simulink model "test_ffts"  (Simulink 6.2)
settings: Solver=ode45  StartTime=0.0  StopTime=300  RelTol=1e-3
undefined symbols (not defined in the file or in its folder): now
libraries: xbsIndex_r3 x1135, fft_library x1, simulink x1
(part 11 of 15)

== system test_ffts/r4_dit_fft/quadplex_bitrev/biplex_bitrev0/bit_reverse ==
  in : Inport  Port=1  LatchInput=off
  bit0 : xbsIndex_r3/Slice  mode=Lower Bit Location + Width  nbits=1  bit1=0  base1=MSB of Input  bit0=0  base0=LSB of Input  boolean_output=off  explicit_period=off  period=1  dbl_ovrd=off
  bit1 : xbsIndex_r3/Slice  mode=Lower Bit Location + Width  nbits=1  bit1=0  base1=MSB of Input  bit0=1  base0=LSB of Input  boolean_output=off  explicit_period=off  period=1  dbl_ovrd=off
  bit2 : xbsIndex_r3/Slice  mode=Lower Bit Location + Width  nbits=1  bit1=0  base1=MSB of Input  bit0=2  base0=LSB of Input  boolean_output=off  explicit_period=off  period=1  dbl_ovrd=off
  bit3 : xbsIndex_r3/Slice  mode=Lower Bit Location + Width  nbits=1  bit1=0  base1=MSB of Input  bit0=3  base0=LSB of Input  boolean_output=off  explicit_period=off  period=1  dbl_ovrd=off
  concat : xbsIndex_r3/Concat  num_inputs=4  explicit_period=off  period=1  dbl_ovrd=off
  out : Outport
  wires:
  in/1 -> bit3/1, bit2/1, bit1/1, bit0/1
  bit3/1 -> concat/4
  bit2/1 -> concat/3
  bit1/1 -> concat/2
  bit0/1 -> concat/1
  concat/1 -> out/1

== system test_ffts/r4_dit_fft/quadplex_bitrev/biplex_bitrev0/c_to_ri ==
  c : Inport  Port=1  LatchInput=off
  force_im : xbsIndex_r3/Reinterpret  force_arith_type=on  arith_type="Signed  (2's comp)"  force_bin_pt=on  bin_pt=0  force_valid=on
  force_re : xbsIndex_r3/Reinterpret  force_arith_type=on  arith_type="Signed  (2's comp)"  force_bin_pt=on  bin_pt=0  force_valid=on
  slice_im : xbsIndex_r3/Slice  mode=Lower Bit Location + Width  nbits=14  bit1=0  base1=MSB of Input  bit0=0  base0=LSB of Input  boolean_output=off  explicit_period=off  period=1  dbl_ovrd=off
  slice_re : xbsIndex_r3/Slice  mode=Upper Bit Location + Width  nbits=14  bit1=0  base1=MSB of Input  bit0=0  base0=LSB of Input  boolean_output=off  explicit_period=off  period=1  dbl_ovrd=off
  re : Outport
  im : Outport  Port=2
  wires:
  slice_re/1 -> force_re/1
  slice_im/1 -> force_im/1
  force_re/1 -> re/1
  force_im/1 -> im/1
  c/1 -> slice_re/1, slice_im/1

== system test_ffts/r4_dit_fft/quadplex_bitrev/biplex_bitrev0/c_to_ri1 ==
  c : Inport  Port=1  LatchInput=off
  force_im : xbsIndex_r3/Reinterpret  force_arith_type=on  arith_type="Signed  (2's comp)"  force_bin_pt=on  bin_pt=0  force_valid=on
  force_re : xbsIndex_r3/Reinterpret  force_arith_type=on  arith_type="Signed  (2's comp)"  force_bin_pt=on  bin_pt=0  force_valid=on
  slice_im : xbsIndex_r3/Slice  mode=Lower Bit Location + Width  nbits=14  bit1=0  base1=MSB of Input  bit0=0  base0=LSB of Input  boolean_output=off  explicit_period=off  period=1  dbl_ovrd=off
  slice_re : xbsIndex_r3/Slice  mode=Upper Bit Location + Width  nbits=14  bit1=0  base1=MSB of Input  bit0=0  base0=LSB of Input  boolean_output=off  explicit_period=off  period=1  dbl_ovrd=off
  re : Outport
  im : Outport  Port=2
  wires:
  slice_re/1 -> force_re/1
  slice_im/1 -> force_im/1
  force_re/1 -> re/1
  force_im/1 -> im/1
  c/1 -> slice_re/1, slice_im/1

== system test_ffts/r4_dit_fft/quadplex_bitrev/biplex_bitrev0/ri_to_c ==
  re : Inport  Port=1  LatchInput=off
  im : Inport  Port=2  LatchInput=off
  concat : xbsIndex_r3/Concat  num_inputs=2  explicit_period=off  period=1  dbl_ovrd=off
  force_im : xbsIndex_r3/Reinterpret  force_arith_type=on  arith_type=Unsigned  force_bin_pt=on  bin_pt=0  force_valid=on
  force_re : xbsIndex_r3/Reinterpret  force_arith_type=on  arith_type=Unsigned  force_bin_pt=on  bin_pt=0  force_valid=on
  c : Outport
  wires:
  force_re/1 -> concat/1
  force_im/1 -> concat/2
  re/1 -> force_re/1
  concat/1 -> c/1
  im/1 -> force_im/1

== system test_ffts/r4_dit_fft/quadplex_bitrev/biplex_bitrev0/ri_to_c1 ==
  re : Inport  Port=1  LatchInput=off
  im : Inport  Port=2  LatchInput=off
  concat : xbsIndex_r3/Concat  num_inputs=2  explicit_period=off  period=1  dbl_ovrd=off
  force_im : xbsIndex_r3/Reinterpret  force_arith_type=on  arith_type=Unsigned  force_bin_pt=on  bin_pt=0  force_valid=on
  force_re : xbsIndex_r3/Reinterpret  force_arith_type=on  arith_type=Unsigned  force_bin_pt=on  bin_pt=0  force_valid=on
  c : Outport
  wires:
  force_re/1 -> concat/1
  force_im/1 -> concat/2
  re/1 -> force_re/1
  concat/1 -> c/1
  im/1 -> force_im/1

== system test_ffts/r4_dit_fft/quadplex_bitrev/biplex_bitrev1/bit_reverse ==
  in : Inport  Port=1  LatchInput=off
  bit0 : xbsIndex_r3/Slice  mode=Lower Bit Location + Width  nbits=1  bit1=0  base1=MSB of Input  bit0=0  base0=LSB of Input  boolean_output=off  explicit_period=off  period=1  dbl_ovrd=off
  bit1 : xbsIndex_r3/Slice  mode=Lower Bit Location + Width  nbits=1  bit1=0  base1=MSB of Input  bit0=1  base0=LSB of Input  boolean_output=off  explicit_period=off  period=1  dbl_ovrd=off
  bit2 : xbsIndex_r3/Slice  mode=Lower Bit Location + Width  nbits=1  bit1=0  base1=MSB of Input  bit0=2  base0=LSB of Input  boolean_output=off  explicit_period=off  period=1  dbl_ovrd=off
  bit3 : xbsIndex_r3/Slice  mode=Lower Bit Location + Width  nbits=1  bit1=0  base1=MSB of Input  bit0=3  base0=LSB of Input  boolean_output=off  explicit_period=off  period=1  dbl_ovrd=off
  concat : xbsIndex_r3/Concat  num_inputs=4  explicit_period=off  period=1  dbl_ovrd=off
  out : Outport
  wires:
  in/1 -> bit3/1, bit2/1, bit1/1, bit0/1
  bit3/1 -> concat/4
  bit2/1 -> concat/3
  bit1/1 -> concat/2
  bit0/1 -> concat/1
  concat/1 -> out/1

== system test_ffts/r4_dit_fft/quadplex_bitrev/biplex_bitrev1/c_to_ri ==
  c : Inport  Port=1  LatchInput=off
  force_im : xbsIndex_r3/Reinterpret  force_arith_type=on  arith_type="Signed  (2's comp)"  force_bin_pt=on  bin_pt=0  force_valid=on
  force_re : xbsIndex_r3/Reinterpret  force_arith_type=on  arith_type="Signed  (2's comp)"  force_bin_pt=on  bin_pt=0  force_valid=on
  slice_im : xbsIndex_r3/Slice  mode=Lower Bit Location + Width  nbits=14  bit1=0  base1=MSB of Input  bit0=0  base0=LSB of Input  boolean_output=off  explicit_period=off  period=1  dbl_ovrd=off
  slice_re : xbsIndex_r3/Slice  mode=Upper Bit Location + Width  nbits=14  bit1=0  base1=MSB of Input  bit0=0  base0=LSB of Input  boolean_output=off  explicit_period=off  period=1  dbl_ovrd=off
  re : Outport
  im : Outport  Port=2
  wires:
  slice_re/1 -> force_re/1
  slice_im/1 -> force_im/1
  force_re/1 -> re/1
  force_im/1 -> im/1
  c/1 -> slice_re/1, slice_im/1

== system test_ffts/r4_dit_fft/quadplex_bitrev/biplex_bitrev1/c_to_ri1 ==
  c : Inport  Port=1  LatchInput=off
  force_im : xbsIndex_r3/Reinterpret  force_arith_type=on  arith_type="Signed  (2's comp)"  force_bin_pt=on  bin_pt=0  force_valid=on
  force_re : xbsIndex_r3/Reinterpret  force_arith_type=on  arith_type="Signed  (2's comp)"  force_bin_pt=on  bin_pt=0  force_valid=on
  slice_im : xbsIndex_r3/Slice  mode=Lower Bit Location + Width  nbits=14  bit1=0  base1=MSB of Input  bit0=0  base0=LSB of Input  boolean_output=off  explicit_period=off  period=1  dbl_ovrd=off
  slice_re : xbsIndex_r3/Slice  mode=Upper Bit Location + Width  nbits=14  bit1=0  base1=MSB of Input  bit0=0  base0=LSB of Input  boolean_output=off  explicit_period=off  period=1  dbl_ovrd=off
  re : Outport
  im : Outport  Port=2
  wires:
  slice_re/1 -> force_re/1
  slice_im/1 -> force_im/1
  force_re/1 -> re/1
  force_im/1 -> im/1
  c/1 -> slice_re/1, slice_im/1

== system test_ffts/r4_dit_fft/quadplex_bitrev/biplex_bitrev1/ri_to_c ==
  re : Inport  Port=1  LatchInput=off
  im : Inport  Port=2  LatchInput=off
  concat : xbsIndex_r3/Concat  num_inputs=2  explicit_period=off  period=1  dbl_ovrd=off
  force_im : xbsIndex_r3/Reinterpret  force_arith_type=on  arith_type=Unsigned  force_bin_pt=on  bin_pt=0  force_valid=on
  force_re : xbsIndex_r3/Reinterpret  force_arith_type=on  arith_type=Unsigned  force_bin_pt=on  bin_pt=0  force_valid=on
  c : Outport
  wires:
  force_re/1 -> concat/1
  force_im/1 -> concat/2
  re/1 -> force_re/1
  concat/1 -> c/1
  im/1 -> force_im/1

== system test_ffts/r4_dit_fft/quadplex_bitrev/biplex_bitrev1/ri_to_c1 ==
  re : Inport  Port=1  LatchInput=off
  im : Inport  Port=2  LatchInput=off
  concat : xbsIndex_r3/Concat  num_inputs=2  explicit_period=off  period=1  dbl_ovrd=off
  force_im : xbsIndex_r3/Reinterpret  force_arith_type=on  arith_type=Unsigned  force_bin_pt=on  bin_pt=0  force_valid=on
  force_re : xbsIndex_r3/Reinterpret  force_arith_type=on  arith_type=Unsigned  force_bin_pt=on  bin_pt=0  force_valid=on
  c : Outport
  wires:
  force_re/1 -> concat/1
  force_im/1 -> concat/2
  re/1 -> force_re/1
  concat/1 -> c/1
  im/1 -> force_im/1

== system test_ffts/r4_dit_fft/quadplex_commutator/biplex_commutator_01/delay_b ==
  in : Inport  Port=1  LatchInput=off
  slr : xbsIndex_r3/Delay  latency=16  reg_retiming=off  explicit_period=off  period=1  en=off  accept_only_valid=off  init_zero=on  dbl_ovrd=off  show_param=off
      settings: xl_area=[0, 0, 0, 0, 0, 0, 0]
  out : Outport
  wires:
  slr/1 -> out/1
  in/1 -> slr/1

== system test_ffts/r4_dit_fft/quadplex_commutator/biplex_commutator_01/delay_lo ==
  in : Inport  Port=1  LatchInput=off
  slr : xbsIndex_r3/Delay  latency=16  reg_retiming=off  explicit_period=off  period=1  en=off  accept_only_valid=off  init_zero=on  dbl_ovrd=off  show_param=off
      settings: xl_area=[0, 0, 0, 0, 0, 0, 0]
  out : Outport
  wires:
  slr/1 -> out/1
  in/1 -> slr/1

== system test_ffts/r4_dit_fft/quadplex_commutator/biplex_commutator_23/delay_b ==
  in : Inport  Port=1  LatchInput=off
  slr : xbsIndex_r3/Delay  latency=16  reg_retiming=off  explicit_period=off  period=1  en=off  accept_only_valid=off  init_zero=on  dbl_ovrd=off  show_param=off
      settings: xl_area=[0, 0, 0, 0, 0, 0, 0]
  out : Outport
  wires:
  slr/1 -> out/1
  in/1 -> slr/1

== system test_ffts/r4_dit_fft/quadplex_commutator/biplex_commutator_23/delay_lo ==
  in : Inport  Port=1  LatchInput=off
  slr : xbsIndex_r3/Delay  latency=16  reg_retiming=off  explicit_period=off  period=1  en=off  accept_only_valid=off  init_zero=on  dbl_ovrd=off  show_param=off
      settings: xl_area=[0, 0, 0, 0, 0, 0, 0]
  out : Outport
  wires:
  slr/1 -> out/1
  in/1 -> slr/1

== system test_ffts/r4_dit_fft/quadplex_commutator/biplex_commutator_ac/delay_b ==
  in : Inport  Port=1  LatchInput=off
  slr : xbsIndex_r3/Delay  latency=32  reg_retiming=off  explicit_period=off  period=1  en=off  accept_only_valid=off  init_zero=on  dbl_ovrd=off  show_param=off
      settings: xl_area=[0, 0, 0, 0, 0, 0, 0]
  out : Outport
  wires:
  slr/1 -> out/1
  in/1 -> slr/1

== system test_ffts/r4_dit_fft/quadplex_commutator/biplex_commutator_ac/delay_lo ==
  in : Inport  Port=1  LatchInput=off
  slr : xbsIndex_r3/Delay  latency=32  reg_retiming=off  explicit_period=off  period=1  en=off  accept_only_valid=off  init_zero=on  dbl_ovrd=off  show_param=off
      settings: xl_area=[0, 0, 0, 0, 0, 0, 0]
  out : Outport
  wires:
  slr/1 -> out/1
  in/1 -> slr/1

== system test_ffts/r4_dit_fft/quadplex_commutator/biplex_commutator_bd/delay_b ==
  in : Inport  Port=1  LatchInput=off
  slr : xbsIndex_r3/Delay  latency=32  reg_retiming=off  explicit_period=off  period=1  en=off  accept_only_valid=off  init_zero=on  dbl_ovrd=off  show_param=off
      settings: xl_area=[0, 0, 0, 0, 0, 0, 0]
  out : Outport
  wires:
  slr/1 -> out/1
  in/1 -> slr/1

== system test_ffts/r4_dit_fft/quadplex_commutator/biplex_commutator_bd/delay_lo ==
  in : Inport  Port=1  LatchInput=off
  slr : xbsIndex_r3/Delay  latency=32  reg_retiming=off  explicit_period=off  period=1  en=off  accept_only_valid=off  init_zero=on  dbl_ovrd=off  show_param=off
      settings: xl_area=[0, 0, 0, 0, 0, 0, 0]
  out : Outport
  wires:
  slr/1 -> out/1
  in/1 -> slr/1

== system test_ffts/r4_dit_fft/r4_dit_stage_1/quadplex_commutator/biplex_commutator_01 ==
  AloAhi : Inport  Port=1  LatchInput=off
  BloBhi : Inport  Port=2  LatchInput=off
  sync_in : Inport  Port=3  LatchInput=off
  Counter : xbsIndex_r3/Counter  cnt_type=Free Running  n_bits=5  bin_pt=0  arith_type=Unsigned  start_count=0  cnt_to=Inf  cnt_by_val=1  operation=Up  explicit_period=off  period=1  load_pin=off  rst=on  en=off  dbl_ovrd=off  show_param=off  use_rpm=on  gen_core=off
      settings: xl_area=[0, 0, 0, 0, 0, 0, 0]
  Delay : xbsIndex_r3/Delay  latency=17  reg_retiming=off  explicit_period=off  period=1  en=off  accept_only_valid=off  init_zero=on  dbl_ovrd=off  show_param=off
      settings: xl_area=[0, 0, 0, 0, 0, 0, 0]
  Mux : xbsIndex_r3/Mux  inputs=2  precision=Full  arith_type="Signed  (2's comp)"  n_bits=8  bin_pt=2  quantization=Truncate  overflow=Wrap  latency=1  explicit_period=off  period=1  en=off  dbl_ovrd=off  show_param=off  mux_type=off  use_rpm=off  gen_core=off
      settings: xl_area=[0, 0, 0, 0, 0, 0, 0]
  Mux1 : xbsIndex_r3/Mux  inputs=2  precision=Full  arith_type="Signed  (2's comp)"  n_bits=8  bin_pt=2  quantization=Truncate  overflow=Wrap  latency=1  explicit_period=off  period=1  en=off  dbl_ovrd=off  show_param=on  mux_type=off  use_rpm=off  gen_core=off
      settings: xl_area=[0, 0, 0, 0, 0, 0, 0]
  delay_b : Subsystem  mask(SLR16 Delay){delay_depth=16}
      mask prompts: delay_depth "Delay Depth"
      mask help: A delay block that uses SLR16 elements for its storage.
      settings: AttributesFormatString=slr depth = 16
      mask Help:
      | <pre>
      | Description::
      | 
      | A delay block that uses SLR16 elements for its storage.
      | 
      | Mask Parameters::
      | 
      | Delay Depth (delay_depth): The length of the delay.
      | </pre>
  delay_lo : Subsystem  mask(SLR16 Delay){delay_depth=16}
      mask prompts: delay_depth "Delay Depth"
      mask help: A delay block that uses SLR16 elements for its storage.
      settings: AttributesFormatString=slr depth = 16
      mask Help:
      | <pre>
      | Description::
      | 
      | A delay block that uses SLR16 elements for its storage.
      | 
      | Mask Parameters::
      | 
      | Delay Depth (delay_depth): The length of the delay.
      | </pre>
  top_bit : xbsIndex_r3/Slice  mode=Upper Bit Location + Width  nbits=1  bit1=0  base1=MSB of Input  bit0=0  base0=LSB of Input  boolean_output=off  explicit_period=off  period=1  dbl_ovrd=off
  AloBlo : Outport
  AhiBhi : Outport  Port=2
  sync_out : Outport  Port=3
  wires:
  Delay/1 -> sync_out/1
  delay_lo/1(out) -> AloBlo/1
  Mux/1 -> delay_lo/1(in)
  delay_b/1(out) -> Mux/3, Mux1/2
  BloBhi/1 -> delay_b/1(in)
  Mux1/1 -> AhiBhi/1
  AloAhi/1 -> Mux1/3, Mux/2
  top_bit/1 -> Mux/1, Mux1/1
  Counter/1 -> top_bit/1
  sync_in/1 -> Delay/1, Counter/1

== system test_ffts/r4_dit_fft/r4_dit_stage_1/quadplex_commutator/biplex_commutator_23 ==
  AloAhi : Inport  Port=1  LatchInput=off
  BloBhi : Inport  Port=2  LatchInput=off
  sync_in : Inport  Port=3  LatchInput=off
  Counter : xbsIndex_r3/Counter  cnt_type=Free Running  n_bits=5  bin_pt=0  arith_type=Unsigned  start_count=0  cnt_to=Inf  cnt_by_val=1  operation=Up  explicit_period=off  period=1  load_pin=off  rst=on  en=off  dbl_ovrd=off  show_param=off  use_rpm=on  gen_core=off
      settings: xl_area=[0, 0, 0, 0, 0, 0, 0]
  Delay : xbsIndex_r3/Delay  latency=17  reg_retiming=off  explicit_period=off  period=1  en=off  accept_only_valid=off  init_zero=on  dbl_ovrd=off  show_param=off
      settings: xl_area=[0, 0, 0, 0, 0, 0, 0]
  Mux : xbsIndex_r3/Mux  inputs=2  precision=Full  arith_type="Signed  (2's comp)"  n_bits=8  bin_pt=2  quantization=Truncate  overflow=Wrap  latency=1  explicit_period=off  period=1  en=off  dbl_ovrd=off  show_param=off  mux_type=off  use_rpm=off  gen_core=off
      settings: xl_area=[0, 0, 0, 0, 0, 0, 0]
  Mux1 : xbsIndex_r3/Mux  inputs=2  precision=Full  arith_type="Signed  (2's comp)"  n_bits=8  bin_pt=2  quantization=Truncate  overflow=Wrap  latency=1  explicit_period=off  period=1  en=off  dbl_ovrd=off  show_param=on  mux_type=off  use_rpm=off  gen_core=off
      settings: xl_area=[0, 0, 0, 0, 0, 0, 0]
  delay_b : Subsystem  mask(SLR16 Delay){delay_depth=16}
      mask prompts: delay_depth "Delay Depth"
      mask help: A delay block that uses SLR16 elements for its storage.
      settings: AttributesFormatString=slr depth = 16
      mask Help:
      | <pre>
      | Description::
      | 
      | A delay block that uses SLR16 elements for its storage.
      | 
      | Mask Parameters::
      | 
      | Delay Depth (delay_depth): The length of the delay.
      | </pre>
  delay_lo : Subsystem  mask(SLR16 Delay){delay_depth=16}
      mask prompts: delay_depth "Delay Depth"
      mask help: A delay block that uses SLR16 elements for its storage.
      settings: AttributesFormatString=slr depth = 16
      mask Help:
      | <pre>
      | Description::
      | 
      | A delay block that uses SLR16 elements for its storage.
      | 
      | Mask Parameters::
      | 
      | Delay Depth (delay_depth): The length of the delay.
      | </pre>
  top_bit : xbsIndex_r3/Slice  mode=Upper Bit Location + Width  nbits=1  bit1=0  base1=MSB of Input  bit0=0  base0=LSB of Input  boolean_output=off  explicit_period=off  period=1  dbl_ovrd=off
  AloBlo : Outport
  AhiBhi : Outport  Port=2
  sync_out : Outport  Port=3
  wires:
  Delay/1 -> sync_out/1
  delay_lo/1(out) -> AloBlo/1
  Mux/1 -> delay_lo/1(in)
  delay_b/1(out) -> Mux/3, Mux1/2
  BloBhi/1 -> delay_b/1(in)
  Mux1/1 -> AhiBhi/1
  AloAhi/1 -> Mux1/3, Mux/2
  top_bit/1 -> Mux/1, Mux1/1
  Counter/1 -> top_bit/1
  sync_in/1 -> Delay/1, Counter/1

== system test_ffts/r4_dit_fft/r4_dit_stage_1/quadplex_commutator/biplex_commutator_ac ==
  AloAhi : Inport  Port=1  LatchInput=off
  BloBhi : Inport  Port=2  LatchInput=off
  sync_in : Inport  Port=3  LatchInput=off
  Counter : xbsIndex_r3/Counter  cnt_type=Free Running  n_bits=6  bin_pt=0  arith_type=Unsigned  start_count=0  cnt_to=Inf  cnt_by_val=1  operation=Up  explicit_period=off  period=1  load_pin=off  rst=on  en=off  dbl_ovrd=off  show_param=off  use_rpm=on  gen_core=off
      settings: xl_area=[0, 0, 0, 0, 0, 0, 0]
  Delay : xbsIndex_r3/Delay  latency=33  reg_retiming=off  explicit_period=off  period=1  en=off  accept_only_valid=off  init_zero=on  dbl_ovrd=off  show_param=off
      settings: xl_area=[0, 0, 0, 0, 0, 0, 0]
  Mux : xbsIndex_r3/Mux  inputs=2  precision=Full  arith_type="Signed  (2's comp)"  n_bits=8  bin_pt=2  quantization=Truncate  overflow=Wrap  latency=1  explicit_period=off  period=1  en=off  dbl_ovrd=off  show_param=off  mux_type=off  use_rpm=off  gen_core=off
      settings: xl_area=[0, 0, 0, 0, 0, 0, 0]
  Mux1 : xbsIndex_r3/Mux  inputs=2  precision=Full  arith_type="Signed  (2's comp)"  n_bits=8  bin_pt=2  quantization=Truncate  overflow=Wrap  latency=1  explicit_period=off  period=1  en=off  dbl_ovrd=off  show_param=on  mux_type=off  use_rpm=off  gen_core=off
      settings: xl_area=[0, 0, 0, 0, 0, 0, 0]
  delay_b : Subsystem  mask(SLR16 Delay){delay_depth=32}
      mask prompts: delay_depth "Delay Depth"
      mask help: A delay block that uses SLR16 elements for its storage.
      settings: AttributesFormatString=slr depth = 32
      mask Help:
      | <pre>
      | Description::
      | 
      | A delay block that uses SLR16 elements for its storage.
      | 
      | Mask Parameters::
      | 
      | Delay Depth (delay_depth): The length of the delay.
      | </pre>
  delay_lo : Subsystem  mask(SLR16 Delay){delay_depth=32}
      mask prompts: delay_depth "Delay Depth"
      mask help: A delay block that uses SLR16 elements for its storage.
      settings: AttributesFormatString=slr depth = 32
      mask Help:
      | <pre>
      | Description::
      | 
      | A delay block that uses SLR16 elements for its storage.
      | 
      | Mask Parameters::
      | 
      | Delay Depth (delay_depth): The length of the delay.
      | </pre>
  top_bit : xbsIndex_r3/Slice  mode=Upper Bit Location + Width  nbits=1  bit1=0  base1=MSB of Input  bit0=0  base0=LSB of Input  boolean_output=off  explicit_period=off  period=1  dbl_ovrd=off
  AloBlo : Outport
  AhiBhi : Outport  Port=2
  sync_out : Outport  Port=3
  wires:
  Delay/1 -> sync_out/1
  delay_lo/1(out) -> AloBlo/1
  Mux/1 -> delay_lo/1(in)
  delay_b/1(out) -> Mux/3, Mux1/2
  BloBhi/1 -> delay_b/1(in)
  Mux1/1 -> AhiBhi/1
  AloAhi/1 -> Mux1/3, Mux/2
  top_bit/1 -> Mux/1, Mux1/1
  Counter/1 -> top_bit/1
  sync_in/1 -> Delay/1, Counter/1

== system test_ffts/r4_dit_fft/r4_dit_stage_1/quadplex_commutator/biplex_commutator_bd ==
  AloAhi : Inport  Port=1  LatchInput=off
  BloBhi : Inport  Port=2  LatchInput=off
  sync_in : Inport  Port=3  LatchInput=off
  Counter : xbsIndex_r3/Counter  cnt_type=Free Running  n_bits=6  bin_pt=0  arith_type=Unsigned  start_count=0  cnt_to=Inf  cnt_by_val=1  operation=Up  explicit_period=off  period=1  load_pin=off  rst=on  en=off  dbl_ovrd=off  show_param=off  use_rpm=on  gen_core=off
      settings: xl_area=[0, 0, 0, 0, 0, 0, 0]
  Delay : xbsIndex_r3/Delay  latency=33  reg_retiming=off  explicit_period=off  period=1  en=off  accept_only_valid=off  init_zero=on  dbl_ovrd=off  show_param=off
      settings: xl_area=[0, 0, 0, 0, 0, 0, 0]
  Mux : xbsIndex_r3/Mux  inputs=2  precision=Full  arith_type="Signed  (2's comp)"  n_bits=8  bin_pt=2  quantization=Truncate  overflow=Wrap  latency=1  explicit_period=off  period=1  en=off  dbl_ovrd=off  show_param=off  mux_type=off  use_rpm=off  gen_core=off
      settings: xl_area=[0, 0, 0, 0, 0, 0, 0]
  Mux1 : xbsIndex_r3/Mux  inputs=2  precision=Full  arith_type="Signed  (2's comp)"  n_bits=8  bin_pt=2  quantization=Truncate  overflow=Wrap  latency=1  explicit_period=off  period=1  en=off  dbl_ovrd=off  show_param=on  mux_type=off  use_rpm=off  gen_core=off
      settings: xl_area=[0, 0, 0, 0, 0, 0, 0]
  delay_b : Subsystem  mask(SLR16 Delay){delay_depth=32}
      mask prompts: delay_depth "Delay Depth"
      mask help: A delay block that uses SLR16 elements for its storage.
      settings: AttributesFormatString=slr depth = 32
      mask Help:
      | <pre>
      | Description::
      | 
      | A delay block that uses SLR16 elements for its storage.
      | 
      | Mask Parameters::
      | 
      | Delay Depth (delay_depth): The length of the delay.
      | </pre>
  delay_lo : Subsystem  mask(SLR16 Delay){delay_depth=32}
      mask prompts: delay_depth "Delay Depth"
      mask help: A delay block that uses SLR16 elements for its storage.
      settings: AttributesFormatString=slr depth = 32
      mask Help:
      | <pre>
      | Description::
      | 
      | A delay block that uses SLR16 elements for its storage.
      | 
      | Mask Parameters::
      | 
      | Delay Depth (delay_depth): The length of the delay.
      | </pre>
  top_bit : xbsIndex_r3/Slice  mode=Upper Bit Location + Width  nbits=1  bit1=0  base1=MSB of Input  bit0=0  base0=LSB of Input  boolean_output=off  explicit_period=off  period=1  dbl_ovrd=off
  AloBlo : Outport
  AhiBhi : Outport  Port=2
  sync_out : Outport  Port=3
  wires:
  Delay/1 -> sync_out/1
  delay_lo/1(out) -> AloBlo/1
  Mux/1 -> delay_lo/1(in)
  delay_b/1(out) -> Mux/3, Mux1/2
  BloBhi/1 -> delay_b/1(in)
  Mux1/1 -> AhiBhi/1
  AloAhi/1 -> Mux1/3, Mux/2
  top_bit/1 -> Mux/1, Mux1/1
  Counter/1 -> top_bit/1
  sync_in/1 -> Delay/1, Counter/1

== system test_ffts/r4_dit_fft/r4_dit_stage_1/r4_butterfly/butterfly0 ==
  a : Inport  Port=1  LatchInput=off
  b : Inport  Port=2  LatchInput=off
  sync_in : Inport  Port=3  LatchInput=off
  Delay : xbsIndex_r3/Delay  latency=1  reg_retiming=off  explicit_period=off  period=1  en=off  accept_only_valid=off  init_zero=on  dbl_ovrd=off  show_param=off
      settings: xl_area=[0, 0, 0, 0, 0, 0, 0]
  add_im : xbsIndex_r3/AddSub  mode=Addition  precision=Full  arith_type=Unsigned  n_bits=8  bin_pt=2  quantization=Truncate  overflow=Wrap  latency=1  explicit_period=off  period=1  use_carryin=off  use_carryout=off  en=off  dbl_ovrd=off  show_param=on  use_core=on  pipeline=on  use_rpm=on  gen_core=off
      settings: xl_area=[0, 0, 0, 0, 0, 0, 0]
  add_re : xbsIndex_r3/AddSub  mode=Addition  precision=Full  arith_type=Unsigned  n_bits=8  bin_pt=2  quantization=Truncate  overflow=Wrap  latency=1  explicit_period=off  period=1  use_carryin=off  use_carryout=off  en=off  dbl_ovrd=off  show_param=on  use_core=on  pipeline=on  use_rpm=on  gen_core=off
      settings: xl_area=[0, 0, 0, 0, 0, 0, 0]
  c_to_ri : Subsystem  mask(Complex to Real-Imag){n_bits=8, bin_pt=0}
      mask prompts: n_bits "Bit Width"; bin_pt "Binary Point"
      mask help: Outputs real and imaginary components of a complex input.
      settings: AttributesFormatString=8_0 r/i
      mask Help:
      | <pre>
      | Description::
      | 
      | Outputs real and imaginary components of a complex input.
      | Useful for simplifying interconnects.
      | See also: Real-Imag to Complex (ri_to_c)
      | 
      | Mask Parameters::
      | 
      | Bit Width (n_bits): Specifies the width of the real/imaginary components.
      | Assumed equal for both components.
      | 
      | Binary Point (bin_pt): Specifies the binary point location in the real/imaginary components.
      | Assumed equal for both components.
      | </pre>
  c_to_ri1 : Subsystem  mask(Complex to Real-Imag){n_bits=8, bin_pt=0}
      mask prompts: n_bits "Bit Width"; bin_pt "Binary Point"
      mask help: Outputs real and imaginary components of a complex input.
      settings: AttributesFormatString=8_0 r/i
      mask Help:
      | <pre>
      | Description::
      | 
      | Outputs real and imaginary components of a complex input.
      | Useful for simplifying interconnects.
      | See also: Real-Imag to Complex (ri_to_c)
      | 
      | Mask Parameters::
      | 
      | Bit Width (n_bits): Specifies the width of the real/imaginary components.
      | Assumed equal for both components.
      | 
      | Binary Point (bin_pt): Specifies the binary point location in the real/imaginary components.
      | Assumed equal for both components.
      | </pre>
  requant{0..3} (4 alike) : xbsIndex_r3/Convert  arith_type="Signed  (2's comp)"  n_bits=9  bin_pt=0  quantization=Truncate  overflow=Wrap  latency=0  explicit_period=off  period=1  dbl_ovrd=off  show_param=on  inserted_by_tool=off  pipeline=on
      settings: xl_area=[0, 0, 0, 0, 0, 0, 0]
  ri_to_c : Subsystem
      mask Type: Real-Imag to Complex
      mask Description: Concatenates real and imaginary inputs into a complex output.
      mask Help:
      | <pre>
      | Description::
      | 
      | Concatenates a real and imaginary input into a complex output.
      | Useful for simplifying interconnects.
      | See also: Complex to Real-Imag (c_to_ri)
      | 
      | Mask Parameters::
      | 
      | (N/A)
      | </pre>
  ri_to_c1 : Subsystem
      mask Type: Real-Imag to Complex
      mask Description: Concatenates real and imaginary inputs into a complex output.
      mask Help:
      | <pre>
      | Description::
      | 
      | Concatenates a real and imaginary input into a complex output.
      | Useful for simplifying interconnects.
      | See also: Complex to Real-Imag (c_to_ri)
      | 
      | Mask Parameters::
      | 
      | (N/A)
      | </pre>
  shift{0..3} (4 alike) : xbsIndex_r3/Scale  scale_factor=0  explicit_period=off  period=1  dbl_ovrd=off
  sub_im : xbsIndex_r3/AddSub  mode=Subtraction  precision=Full  arith_type=Unsigned  n_bits=8  bin_pt=2  quantization=Truncate  overflow=Wrap  latency=1  explicit_period=off  period=1  use_carryin=off  use_carryout=off  en=off  dbl_ovrd=off  show_param=on  use_core=on  pipeline=on  use_rpm=on  gen_core=off
      settings: xl_area=[0, 0, 0, 0, 0, 0, 0]
  sub_re : xbsIndex_r3/AddSub  mode=Subtraction  precision=Full  arith_type=Unsigned  n_bits=8  bin_pt=2  quantization=Truncate  overflow=Wrap  latency=1  explicit_period=off  period=1  use_carryin=off  use_carryout=off  en=off  dbl_ovrd=off  show_param=on  use_core=on  pipeline=on  use_rpm=on  gen_core=off
      settings: xl_area=[0, 0, 0, 0, 0, 0, 0]
  a+b : Outport
  a-b : Outport  Port=2
  sync_out : Outport  Port=3
  wires:
  shift3/1 -> requant3/1
  sub_im/1 -> shift3/1
  shift2/1 -> requant2/1
  sub_re/1 -> shift2/1
  shift1/1 -> requant1/1
  shift0/1 -> requant0/1
  requant3/1 -> ri_to_c1/2(im)
  requant2/1 -> ri_to_c1/1(re)
  requant1/1 -> ri_to_c/2(im)
  requant0/1 -> ri_to_c/1(re)
  Delay/1 -> sync_out/1
  sync_in/1 -> Delay/1
  ri_to_c1/1(c) -> a-b/1
  ri_to_c/1(c) -> a+b/1
  add_im/1 -> shift1/1
  add_re/1 -> shift0/1
  a/1 -> c_to_ri/1(c)
  c_to_ri/2(im) -> sub_im/1, add_im/1
  c_to_ri/1(re) -> sub_re/1, add_re/1
  c_to_ri1/2(im) -> add_im/2, sub_im/2
  c_to_ri1/1(re) -> add_re/2, sub_re/2
  b/1 -> c_to_ri1/1(c)

== system test_ffts/r4_dit_fft/r4_dit_stage_1/r4_butterfly/butterfly1 ==
  a : Inport  Port=1  LatchInput=off
  b : Inport  Port=2  LatchInput=off
  sync_in : Inport  Port=3  LatchInput=off
  Delay : xbsIndex_r3/Delay  latency=1  reg_retiming=off  explicit_period=off  period=1  en=off  accept_only_valid=off  init_zero=on  dbl_ovrd=off  show_param=off
      settings: xl_area=[0, 0, 0, 0, 0, 0, 0]
  add_im : xbsIndex_r3/AddSub  mode=Addition  precision=Full  arith_type=Unsigned  n_bits=8  bin_pt=2  quantization=Truncate  overflow=Wrap  latency=1  explicit_period=off  period=1  use_carryin=off  use_carryout=off  en=off  dbl_ovrd=off  show_param=on  use_core=on  pipeline=on  use_rpm=on  gen_core=off
      settings: xl_area=[0, 0, 0, 0, 0, 0, 0]
  add_re : xbsIndex_r3/AddSub  mode=Addition  precision=Full  arith_type=Unsigned  n_bits=8  bin_pt=2  quantization=Truncate  overflow=Wrap  latency=1  explicit_period=off  period=1  use_carryin=off  use_carryout=off  en=off  dbl_ovrd=off  show_param=on  use_core=on  pipeline=on  use_rpm=on  gen_core=off
      settings: xl_area=[0, 0, 0, 0, 0, 0, 0]
  c_to_ri : Subsystem  mask(Complex to Real-Imag){n_bits=8, bin_pt=0}
      mask prompts: n_bits "Bit Width"; bin_pt "Binary Point"
      mask help: Outputs real and imaginary components of a complex input.
      settings: AttributesFormatString=8_0 r/i
      mask Help:
      | <pre>
      | Description::
      | 
      | Outputs real and imaginary components of a complex input.
      | Useful for simplifying interconnects.
      | See also: Real-Imag to Complex (ri_to_c)
      | 
      | Mask Parameters::
      | 
      | Bit Width (n_bits): Specifies the width of the real/imaginary components.
      | Assumed equal for both components.
      | 
      | Binary Point (bin_pt): Specifies the binary point location in the real/imaginary components.
      | Assumed equal for both components.
      | </pre>
  c_to_ri1 : Subsystem  mask(Complex to Real-Imag){n_bits=8, bin_pt=0}
      mask prompts: n_bits "Bit Width"; bin_pt "Binary Point"
      mask help: Outputs real and imaginary components of a complex input.
      settings: AttributesFormatString=8_0 r/i
      mask Help:
      | <pre>
      | Description::
      | 
      | Outputs real and imaginary components of a complex input.
      | Useful for simplifying interconnects.
      | See also: Real-Imag to Complex (ri_to_c)
      | 
      | Mask Parameters::
      | 
      | Bit Width (n_bits): Specifies the width of the real/imaginary components.
      | Assumed equal for both components.
      | 
      | Binary Point (bin_pt): Specifies the binary point location in the real/imaginary components.
      | Assumed equal for both components.
      | </pre>
  requant{0..3} (4 alike) : xbsIndex_r3/Convert  arith_type="Signed  (2's comp)"  n_bits=9  bin_pt=0  quantization=Truncate  overflow=Wrap  latency=0  explicit_period=off  period=1  dbl_ovrd=off  show_param=on  inserted_by_tool=off  pipeline=on
      settings: xl_area=[0, 0, 0, 0, 0, 0, 0]
  ri_to_c : Subsystem
      mask Type: Real-Imag to Complex
      mask Description: Concatenates real and imaginary inputs into a complex output.
      mask Help:
      | <pre>
      | Description::
      | 
      | Concatenates a real and imaginary input into a complex output.
      | Useful for simplifying interconnects.
      | See also: Complex to Real-Imag (c_to_ri)
      | 
      | Mask Parameters::
      | 
      | (N/A)
      | </pre>
  ri_to_c1 : Subsystem
      mask Type: Real-Imag to Complex
      mask Description: Concatenates real and imaginary inputs into a complex output.
      mask Help:
      | <pre>
      | Description::
      | 
      | Concatenates a real and imaginary input into a complex output.
      | Useful for simplifying interconnects.
      | See also: Complex to Real-Imag (c_to_ri)
      | 
      | Mask Parameters::
      | 
      | (N/A)
      | </pre>
  shift{0..3} (4 alike) : xbsIndex_r3/Scale  scale_factor=0  explicit_period=off  period=1  dbl_ovrd=off
  sub_im : xbsIndex_r3/AddSub  mode=Subtraction  precision=Full  arith_type=Unsigned  n_bits=8  bin_pt=2  quantization=Truncate  overflow=Wrap  latency=1  explicit_period=off  period=1  use_carryin=off  use_carryout=off  en=off  dbl_ovrd=off  show_param=on  use_core=on  pipeline=on  use_rpm=on  gen_core=off
      settings: xl_area=[0, 0, 0, 0, 0, 0, 0]
  sub_re : xbsIndex_r3/AddSub  mode=Subtraction  precision=Full  arith_type=Unsigned  n_bits=8  bin_pt=2  quantization=Truncate  overflow=Wrap  latency=1  explicit_period=off  period=1  use_carryin=off  use_carryout=off  en=off  dbl_ovrd=off  show_param=on  use_core=on  pipeline=on  use_rpm=on  gen_core=off
      settings: xl_area=[0, 0, 0, 0, 0, 0, 0]
  a+b : Outport
  a-b : Outport  Port=2
  sync_out : Outport  Port=3
  wires:
  shift3/1 -> requant3/1
  sub_im/1 -> shift3/1
  shift2/1 -> requant2/1
  sub_re/1 -> shift2/1
  shift1/1 -> requant1/1
  shift0/1 -> requant0/1
  requant3/1 -> ri_to_c1/2(im)
  requant2/1 -> ri_to_c1/1(re)
  requant1/1 -> ri_to_c/2(im)
  requant0/1 -> ri_to_c/1(re)
  Delay/1 -> sync_out/1
  sync_in/1 -> Delay/1
  ri_to_c1/1(c) -> a-b/1
  ri_to_c/1(c) -> a+b/1
  add_im/1 -> shift1/1
  add_re/1 -> shift0/1
  a/1 -> c_to_ri/1(c)
  c_to_ri/2(im) -> sub_im/1, add_im/1
  c_to_ri/1(re) -> sub_re/1, add_re/1
  c_to_ri1/2(im) -> add_im/2, sub_im/2
  c_to_ri1/1(re) -> add_re/2, sub_re/2
  b/1 -> c_to_ri1/1(c)

== system test_ffts/r4_dit_fft/r4_dit_stage_1/r4_butterfly/butterfly2 ==
  a : Inport  Port=1  LatchInput=off
  b : Inport  Port=2  LatchInput=off
  sync_in : Inport  Port=3  LatchInput=off
  Delay : xbsIndex_r3/Delay  latency=1  reg_retiming=off  explicit_period=off  period=1  en=off  accept_only_valid=off  init_zero=on  dbl_ovrd=off  show_param=off
      settings: xl_area=[0, 0, 0, 0, 0, 0, 0]
  add_im : xbsIndex_r3/AddSub  mode=Addition  precision=Full  arith_type=Unsigned  n_bits=8  bin_pt=2  quantization=Truncate  overflow=Wrap  latency=1  explicit_period=off  period=1  use_carryin=off  use_carryout=off  en=off  dbl_ovrd=off  show_param=on  use_core=on  pipeline=on  use_rpm=on  gen_core=off
      settings: xl_area=[0, 0, 0, 0, 0, 0, 0]
  add_re : xbsIndex_r3/AddSub  mode=Addition  precision=Full  arith_type=Unsigned  n_bits=8  bin_pt=2  quantization=Truncate  overflow=Wrap  latency=1  explicit_period=off  period=1  use_carryin=off  use_carryout=off  en=off  dbl_ovrd=off  show_param=on  use_core=on  pipeline=on  use_rpm=on  gen_core=off
      settings: xl_area=[0, 0, 0, 0, 0, 0, 0]
  c_to_ri : Subsystem  mask(Complex to Real-Imag){n_bits=9, bin_pt=0}
      mask prompts: n_bits "Bit Width"; bin_pt "Binary Point"
      mask help: Outputs real and imaginary components of a complex input.
      settings: AttributesFormatString=9_0 r/i
      mask Help:
      | <pre>
      | Description::
      | 
      | Outputs real and imaginary components of a complex input.
      | Useful for simplifying interconnects.
      | See also: Real-Imag to Complex (ri_to_c)
      | 
      | Mask Parameters::
      | 
      | Bit Width (n_bits): Specifies the width of the real/imaginary components.
      | Assumed equal for both components.
      | 
      | Binary Point (bin_pt): Specifies the binary point location in the real/imaginary components.
      | Assumed equal for both components.
      | </pre>
  c_to_ri1 : Subsystem  mask(Complex to Real-Imag){n_bits=9, bin_pt=0}
      mask prompts: n_bits "Bit Width"; bin_pt "Binary Point"
      mask help: Outputs real and imaginary components of a complex input.
      settings: AttributesFormatString=9_0 r/i
      mask Help:
      | <pre>
      | Description::
      | 
      | Outputs real and imaginary components of a complex input.
      | Useful for simplifying interconnects.
      | See also: Real-Imag to Complex (ri_to_c)
      | 
      | Mask Parameters::
      | 
      | Bit Width (n_bits): Specifies the width of the real/imaginary components.
      | Assumed equal for both components.
      | 
      | Binary Point (bin_pt): Specifies the binary point location in the real/imaginary components.
      | Assumed equal for both components.
      | </pre>
  requant{0..3} (4 alike) : xbsIndex_r3/Convert  arith_type="Signed  (2's comp)"  n_bits=10  bin_pt=0  quantization=Truncate  overflow=Wrap  latency=0  explicit_period=off  period=1  dbl_ovrd=off  show_param=on  inserted_by_tool=off  pipeline=on
      settings: xl_area=[0, 0, 0, 0, 0, 0, 0]
  ri_to_c : Subsystem
      mask Type: Real-Imag to Complex
      mask Description: Concatenates real and imaginary inputs into a complex output.
      mask Help:
      | <pre>
      | Description::
      | 
      | Concatenates a real and imaginary input into a complex output.
      | Useful for simplifying interconnects.
      | See also: Complex to Real-Imag (c_to_ri)
      | 
      | Mask Parameters::
      | 
      | (N/A)
      | </pre>
  ri_to_c1 : Subsystem
      mask Type: Real-Imag to Complex
      mask Description: Concatenates real and imaginary inputs into a complex output.
      mask Help:
      | <pre>
      | Description::
      | 
      | Concatenates a real and imaginary input into a complex output.
      | Useful for simplifying interconnects.
      | See also: Complex to Real-Imag (c_to_ri)
      | 
      | Mask Parameters::
      | 
      | (N/A)
      | </pre>
  shift{0..3} (4 alike) : xbsIndex_r3/Scale  scale_factor=0  explicit_period=off  period=1  dbl_ovrd=off
  sub_im : xbsIndex_r3/AddSub  mode=Subtraction  precision=Full  arith_type=Unsigned  n_bits=8  bin_pt=2  quantization=Truncate  overflow=Wrap  latency=1  explicit_period=off  period=1  use_carryin=off  use_carryout=off  en=off  dbl_ovrd=off  show_param=on  use_core=on  pipeline=on  use_rpm=on  gen_core=off
      settings: xl_area=[0, 0, 0, 0, 0, 0, 0]
  sub_re : xbsIndex_r3/AddSub  mode=Subtraction  precision=Full  arith_type=Unsigned  n_bits=8  bin_pt=2  quantization=Truncate  overflow=Wrap  latency=1  explicit_period=off  period=1  use_carryin=off  use_carryout=off  en=off  dbl_ovrd=off  show_param=on  use_core=on  pipeline=on  use_rpm=on  gen_core=off
      settings: xl_area=[0, 0, 0, 0, 0, 0, 0]
  a+b : Outport
  a-b : Outport  Port=2
  sync_out : Outport  Port=3
  wires:
  shift3/1 -> requant3/1
  sub_im/1 -> shift3/1
  shift2/1 -> requant2/1
  sub_re/1 -> shift2/1
  shift1/1 -> requant1/1
  shift0/1 -> requant0/1
  requant3/1 -> ri_to_c1/2(im)
  requant2/1 -> ri_to_c1/1(re)
  requant1/1 -> ri_to_c/2(im)
  requant0/1 -> ri_to_c/1(re)
  Delay/1 -> sync_out/1
  sync_in/1 -> Delay/1
  ri_to_c1/1(c) -> a-b/1
  ri_to_c/1(c) -> a+b/1
  add_im/1 -> shift1/1
  add_re/1 -> shift0/1
  a/1 -> c_to_ri/1(c)
  c_to_ri/2(im) -> sub_im/1, add_im/1
  c_to_ri/1(re) -> sub_re/1, add_re/1
  c_to_ri1/2(im) -> add_im/2, sub_im/2
  c_to_ri1/1(re) -> add_re/2, sub_re/2
  b/1 -> c_to_ri1/1(c)

== system test_ffts/r4_dit_fft/r4_dit_stage_1/r4_butterfly/butterfly3j ==
  a : Inport  Port=1  LatchInput=off
  b : Inport  Port=2  LatchInput=off
  sync_in : Inport  Port=3  LatchInput=off
  Delay : xbsIndex_r3/Delay  latency=1  reg_retiming=off  explicit_period=off  period=1  en=off  accept_only_valid=off  init_zero=on  dbl_ovrd=off  show_param=off
      settings: xl_area=[0, 0, 0, 0, 0, 0, 0]
  add_im : xbsIndex_r3/AddSub  mode=Subtraction  precision=Full  arith_type=Unsigned  n_bits=8  bin_pt=2  quantization=Truncate  overflow=Wrap  latency=1  explicit_period=off  period=1  use_carryin=off  use_carryout=off  en=off  dbl_ovrd=off  show_param=on  use_core=on  pipeline=on  use_rpm=on  gen_core=off
      settings: xl_area=[0, 0, 0, 0, 0, 0, 0]
  add_re : xbsIndex_r3/AddSub  mode=Addition  precision=Full  arith_type=Unsigned  n_bits=8  bin_pt=2  quantization=Truncate  overflow=Wrap  latency=1  explicit_period=off  period=1  use_carryin=off  use_carryout=off  en=off  dbl_ovrd=off  show_param=on  use_core=on  pipeline=on  use_rpm=on  gen_core=off
      settings: xl_area=[0, 0, 0, 0, 0, 0, 0]
  c_to_ri : Subsystem  mask(Complex to Real-Imag){n_bits=9, bin_pt=0}
      mask prompts: n_bits "Bit Width"; bin_pt "Binary Point"
      mask help: Outputs real and imaginary components of a complex input.
      settings: AttributesFormatString=9_0 r/i
      mask Help:
      | <pre>
      | Description::
      | 
      | Outputs real and imaginary components of a complex input.
      | Useful for simplifying interconnects.
      | See also: Real-Imag to Complex (ri_to_c)
      | 
      | Mask Parameters::
      | 
      | Bit Width (n_bits): Specifies the width of the real/imaginary components.
      | Assumed equal for both components.
      | 
      | Binary Point (bin_pt): Specifies the binary point location in the real/imaginary components.
      | Assumed equal for both components.
      | </pre>
  c_to_ri1 : Subsystem  mask(Complex to Real-Imag){n_bits=9, bin_pt=0}
      mask prompts: n_bits "Bit Width"; bin_pt "Binary Point"
      mask help: Outputs real and imaginary components of a complex input.
      settings: AttributesFormatString=9_0 r/i
      mask Help:
      | <pre>
      | Description::
      | 
      | Outputs real and imaginary components of a complex input.
      | Useful for simplifying interconnects.
      | See also: Real-Imag to Complex (ri_to_c)
      | 
      | Mask Parameters::
      | 
      | Bit Width (n_bits): Specifies the width of the real/imaginary components.
      | Assumed equal for both components.
      | 
      | Binary Point (bin_pt): Specifies the binary point location in the real/imaginary components.
      | Assumed equal for both components.
      | </pre>
  requant{0..3} (4 alike) : xbsIndex_r3/Convert  arith_type="Signed  (2's comp)"  n_bits=10  bin_pt=0  quantization=Truncate  overflow=Wrap  latency=0  explicit_period=off  period=1  dbl_ovrd=off  show_param=on  inserted_by_tool=off  pipeline=on
      settings: xl_area=[0, 0, 0, 0, 0, 0, 0]
  ri_to_c : Subsystem
      mask Type: Real-Imag to Complex
      mask Description: Concatenates real and imaginary inputs into a complex output.
      mask Help:
      | <pre>
      | Description::
      | 
      | Concatenates a real and imaginary input into a complex output.
      | Useful for simplifying interconnects.
      | See also: Complex to Real-Imag (c_to_ri)
      | 
      | Mask Parameters::
      | 
      | (N/A)
      | </pre>
  ri_to_c1 : Subsystem
      mask Type: Real-Imag to Complex
      mask Description: Concatenates real and imaginary inputs into a complex output.
      mask Help:
      | <pre>
      | Description::
      | 
      | Concatenates a real and imaginary input into a complex output.
      | Useful for simplifying interconnects.
      | See also: Complex to Real-Imag (c_to_ri)
      | 
      | Mask Parameters::
      | 
      | (N/A)
      | </pre>
  shift{0..3} (4 alike) : xbsIndex_r3/Scale  scale_factor=0  explicit_period=off  period=1  dbl_ovrd=off
  sub_im : xbsIndex_r3/AddSub  mode=Addition  precision=Full  arith_type=Unsigned  n_bits=8  bin_pt=2  quantization=Truncate  overflow=Wrap  latency=1  explicit_period=off  period=1  use_carryin=off  use_carryout=off  en=off  dbl_ovrd=off  show_param=on  use_core=on  pipeline=on  use_rpm=on  gen_core=off
      settings: xl_area=[0, 0, 0, 0, 0, 0, 0]
  sub_re : xbsIndex_r3/AddSub  mode=Subtraction  precision=Full  arith_type=Unsigned  n_bits=8  bin_pt=2  quantization=Truncate  overflow=Wrap  latency=1  explicit_period=off  period=1  use_carryin=off  use_carryout=off  en=off  dbl_ovrd=off  show_param=on  use_core=on  pipeline=on  use_rpm=on  gen_core=off
      settings: xl_area=[0, 0, 0, 0, 0, 0, 0]
  a+b : Outport
  a-b : Outport  Port=2
  sync_out : Outport  Port=3
  wires:
  requant3/1 -> ri_to_c1/2(im)
  requant2/1 -> ri_to_c1/1(re)
  requant1/1 -> ri_to_c/2(im)
  requant0/1 -> ri_to_c/1(re)
  shift3/1 -> requant3/1
  shift2/1 -> requant2/1
  shift1/1 -> requant1/1
  shift0/1 -> requant0/1
  sub_im/1 -> shift3/1
  sub_re/1 -> shift2/1
  b/1 -> c_to_ri1/1(c)
  c_to_ri1/1(re) -> add_im/2, sub_im/2
  c_to_ri1/2(im) -> add_re/2, sub_re/2
  c_to_ri/1(re) -> sub_re/1, add_re/1
  c_to_ri/2(im) -> sub_im/1, add_im/1
  a/1 -> c_to_ri/1(c)
  add_re/1 -> shift0/1
  add_im/1 -> shift1/1
  ri_to_c/1(c) -> a+b/1
  ri_to_c1/1(c) -> a-b/1
  sync_in/1 -> Delay/1
  Delay/1 -> sync_out/1

== system test_ffts/r4_dit_fft/r4_dit_stage_2/quadplex_commutator/biplex_commutator_01 ==
  AloAhi : Inport  Port=1  LatchInput=off
  BloBhi : Inport  Port=2  LatchInput=off
  sync_in : Inport  Port=3  LatchInput=off
  Counter : xbsIndex_r3/Counter  cnt_type=Free Running  n_bits=3  bin_pt=0  arith_type=Unsigned  start_count=0  cnt_to=Inf  cnt_by_val=1  operation=Up  explicit_period=off  period=1  load_pin=off  rst=on  en=off  dbl_ovrd=off  show_param=off  use_rpm=on  gen_core=off
      settings: xl_area=[0, 0, 0, 0, 0, 0, 0]
  Delay : xbsIndex_r3/Delay  latency=5  reg_retiming=off  explicit_period=off  period=1  en=off  accept_only_valid=off  init_zero=on  dbl_ovrd=off  show_param=off
      settings: xl_area=[0, 0, 0, 0, 0, 0, 0]
  Mux : xbsIndex_r3/Mux  inputs=2  precision=Full  arith_type="Signed  (2's comp)"  n_bits=8  bin_pt=2  quantization=Truncate  overflow=Wrap  latency=1  explicit_period=off  period=1  en=off  dbl_ovrd=off  show_param=off  mux_type=off  use_rpm=off  gen_core=off
      settings: xl_area=[0, 0, 0, 0, 0, 0, 0]
  Mux1 : xbsIndex_r3/Mux  inputs=2  precision=Full  arith_type="Signed  (2's comp)"  n_bits=8  bin_pt=2  quantization=Truncate  overflow=Wrap  latency=1  explicit_period=off  period=1  en=off  dbl_ovrd=off  show_param=on  mux_type=off  use_rpm=off  gen_core=off
      settings: xl_area=[0, 0, 0, 0, 0, 0, 0]
  delay_b : Subsystem  mask(SLR16 Delay){delay_depth=4}
      mask prompts: delay_depth "Delay Depth"
      mask help: A delay block that uses SLR16 elements for its storage.
      settings: AttributesFormatString=slr depth = 4
      mask Help:
      | <pre>
      | Description::
      | 
      | A delay block that uses SLR16 elements for its storage.
      | 
      | Mask Parameters::
      | 
      | Delay Depth (delay_depth): The length of the delay.
      | </pre>
  delay_lo : Subsystem  mask(SLR16 Delay){delay_depth=4}
      mask prompts: delay_depth "Delay Depth"
      mask help: A delay block that uses SLR16 elements for its storage.
      settings: AttributesFormatString=slr depth = 4
      mask Help:
      | <pre>
      | Description::
      | 
      | A delay block that uses SLR16 elements for its storage.
      | 
      | Mask Parameters::
      | 
      | Delay Depth (delay_depth): The length of the delay.
      | </pre>
  top_bit : xbsIndex_r3/Slice  mode=Upper Bit Location + Width  nbits=1  bit1=0  base1=MSB of Input  bit0=0  base0=LSB of Input  boolean_output=off  explicit_period=off  period=1  dbl_ovrd=off
  AloBlo : Outport
  AhiBhi : Outport  Port=2
  sync_out : Outport  Port=3
  wires:
  Delay/1 -> sync_out/1
  delay_lo/1(out) -> AloBlo/1
  Mux/1 -> delay_lo/1(in)
  delay_b/1(out) -> Mux/3, Mux1/2
  BloBhi/1 -> delay_b/1(in)
  Mux1/1 -> AhiBhi/1
  AloAhi/1 -> Mux1/3, Mux/2
  top_bit/1 -> Mux/1, Mux1/1
  Counter/1 -> top_bit/1
  sync_in/1 -> Delay/1, Counter/1
